simulink model "Unweighted_Plant_1"  (R2017a)
settings: Solver=VariableStepAuto  StartTime=0.0  StopTime=10.0  RelTol=1e-3
values from neighbouring files (symbols this model uses):
  A_new = zeros(6,6)    [main_1.m]
  B_new = zeros(6,2)    [main_1.m]
  C_new = [1 0 0 0 0 0;0 1 0 0 0 0;0 0 1 0 0 0]    [main_1.m]
  D_new = zeros(3,2)    [main_1.m]
libraries: cstblocks x3
settings Model: Creator=Ali  LastModifiedBy=Ali

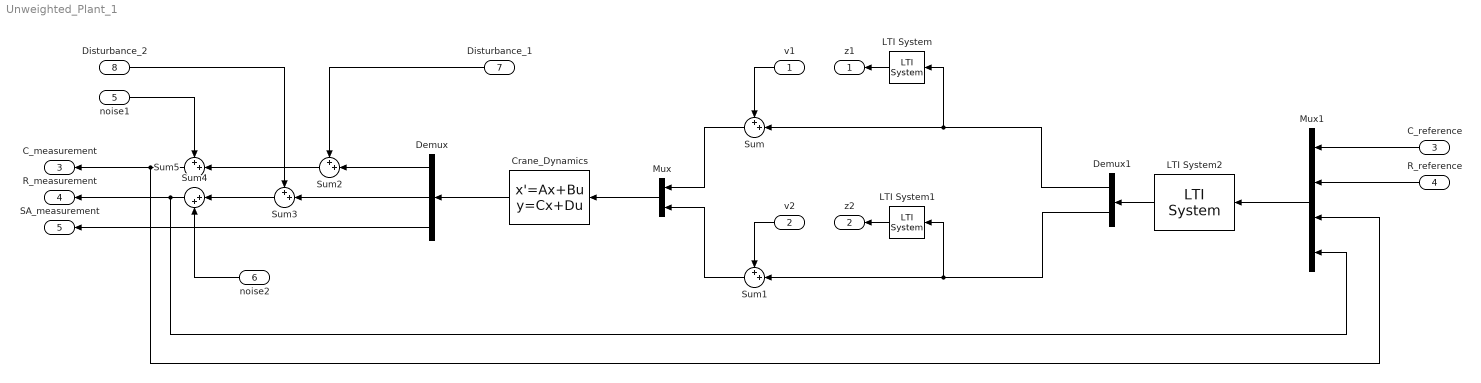
== system Unweighted_Plant_1 ==
  v1 : Inport
  v2 : Inport  Port=2
  C_reference : Inport  Port=3
  R_reference : Inport  Port=4
  noise1 : Inport  Port=5
  noise2 : Inport  Port=6
  Disturbance_1 : Inport  Port=7
  Disturbance_2 : Inport  Port=8
  Crane_Dynamics : StateSpace  A=A_new  B=B_new  C=C_new  D=D_new  X0=0
  Demux : Demux  Outputs=3
  Demux1 : Demux  Outputs=2
  LTI System : cstblocks/LTI System  sys=Wa1  IC=[]
  LTI System1 : cstblocks/LTI System  sys=Wa2  IC=[]
  LTI System2 : cstblocks/LTI System  sys=K  IC=[]
  Mux : Mux  Inputs=2
  Mux1 : Mux
  Sum{,1..3,5} (5 alike) : Sum  Inputs=++|
  Sum4 : Sum  Inputs=|++
  z1 : Outport
  z2 : Outport  Port=2
  C_measurement : Outport  Port=3
  R_measurement : Outport  Port=4
  SA_measurement : Outport  Port=5
  wires:
  noise1/1 -> Sum5/1
  v1/1 -> Sum/1
  Demux1/2 -> LTI System1/1, Sum1/2
  Disturbance_1/1 -> Sum2/1
  LTI System/1 -> z1/1
  Sum3/1 -> Sum4/1
  Disturbance_2/1 -> Sum3/1
  Mux/1 -> Crane_Dynamics/1
  Sum1/1 -> Mux/2
  Crane_Dynamics/1 -> Demux/1
  Demux/2 -> Sum3/2
  LTI System1/1 -> z2/1
  Sum/1 -> Mux/1
  v2/1 -> Sum1/1
  Demux1/1 -> LTI System/1, Sum/2
  noise2/1 -> Sum4/2
  Sum2/1 -> Sum5/2
  Demux/1 -> Sum2/2
  LTI System2/1 -> Demux1/1
  Mux1/1 -> LTI System2/1
  C_reference/1 -> Mux1/1
  R_reference/1 -> Mux1/2
  Sum4/1 -> Mux1/4, R_measurement/1
  Sum5/1 -> C_measurement/1, Mux1/3
  Demux/3 -> SA_measurement/1
